simulink model "lateral_observer"  (R2024b)
settings: Solver=VariableStepAuto  StartTime=0.0  StopTime=time(end)  MaxStep=1E-03  RelTol=1e-3
InitFcn:
  | lateral_observer_init;
values from neighbouring files (symbols this model uses):
  A = sys_struct.E \ sys_struct.A    [kf_design.m]    (also in lateral_observer_init.m = sys.A; observerLMI.m = sys.A; observerLMIHinf.m = sys.A; observerLMIHinfReducedOrder.m = sys.A)
  B = sys_struct.E \ sys_struct.B    [kf_design.m]    (also in lateral_observer_init.m = sys.B(:,2); observerLMI.m = sys.B; observerLMIHinf.m = sys.B; observerLMIHinfReducedOrder.m = sys.B)
  C = [ ... (first row only)    [kf_design.m]    (also in lateral_observer_init.m; observerLMI.m = sys.C; observerLMIHinf.m = sys.C; observerLMIHinfReducedOrder.m = sys.C)
  L = value(P)\value(R)    [lateral_observer_init.m]    (also in observerLMI.m = Pval \ Rval; observerLMIHinf.m = value(P) \ value(R); observerLMIHinfReducedOrder.m = value(P) \ value(R); observerLMIHinfUIO.m = value(P) \ value(R))
  x0 = arrayfun(@(x)x.Data(1),x)    [lateral_observer_init.m]
settings Model: Creator=marti  LastModifiedBy=marti

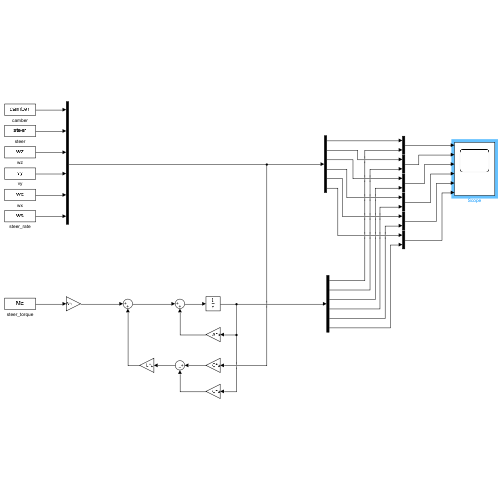
[thumbnail: Simulink's stored preview of the top-level diagram]
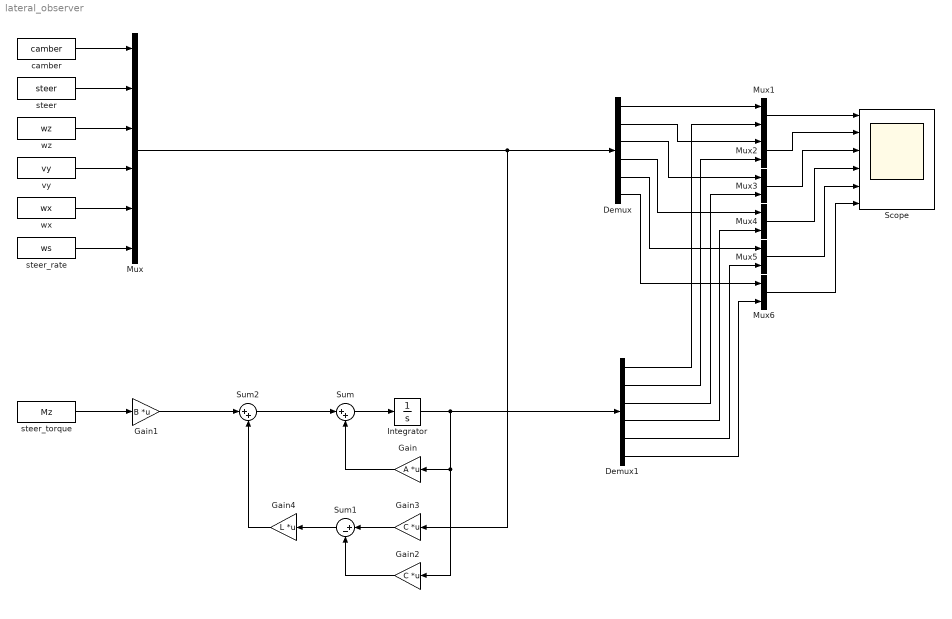
== system lateral_observer ==
  Demux : Demux  Outputs=6
  Demux1 : Demux  Outputs=6
  Gain : Gain  Gain=A  Multiplication=Matrix(K*u)
  Gain1 : Gain  Gain=B  Multiplication=Matrix(K*u)
  Gain2 : Gain  Gain=C  Multiplication=Matrix(K*u)
  Gain3 : Gain  Gain=C  Multiplication=Matrix(K*u)
  Gain4 : Gain  Gain=L  Multiplication=Matrix(K*u)
  Integrator : Integrator  InitialCondition=x0
  Mux : Mux  Inputs=6
  Mux{1..6} (6 alike) : Mux  Inputs=2
  Scope : Scope  NumInputPorts=6
  Sum : Sum  Inputs=|++
  Sum1 : Sum  Inputs=|+-
  Sum2 : Sum  Inputs=|++
  camber : FromWorkspace  VariableName=camber
  steer : FromWorkspace  VariableName=steer
  steer_rate : FromWorkspace  VariableName=ws
  steer_torque : FromWorkspace  VariableName=Mz
  vy : FromWorkspace  VariableName=vy
  wx : FromWorkspace  VariableName=wx
  wz : FromWorkspace  VariableName=wz
  wires:
  camber/1 -> Mux/1
  steer/1 -> Mux/2
  wz/1 -> Mux/3
  vy/1 -> Mux/4
  wx/1 -> Mux/5
  steer_rate/1 -> Mux/6
  Mux/1 -> Gain3/1, Demux/1
  Mux1/1 -> Scope/1
  Mux2/1 -> Scope/2
  Mux3/1 -> Scope/3
  Mux4/1 -> Scope/4
  Mux5/1 -> Scope/5
  Mux6/1 -> Scope/6
  Demux/1 -> Mux1/1
  Demux/2 -> Mux2/1
  Demux/3 -> Mux3/1
  Demux/4 -> Mux4/1
  Demux/5 -> Mux5/1
  Demux/6 -> Mux6/1
  Demux1/6 -> Mux6/2
  Demux1/5 -> Mux5/2
  Demux1/4 -> Mux4/2
  Demux1/3 -> Mux3/2
  Demux1/2 -> Mux2/2
  Demux1/1 -> Mux1/2
  Integrator/1 -> Demux1/1, Gain2/1, Gain/1
  Sum/1 -> Integrator/1
  Gain/1 -> Sum/2
  steer_torque/1 -> Gain1/1
  Gain2/1 -> Sum1/2
  Gain3/1 -> Sum1/1
  Sum1/1 -> Gain4/1
  Sum2/1 -> Sum/1
  Gain4/1 -> Sum2/2
  Gain1/1 -> Sum2/1
